simulink model "progetto_tesi_def"  (R2023b)
settings: Solver=ode1  StartTime=0.0  StopTime=inf  FixedStep=dt  RelTol=1e-3
values from neighbouring files (symbols this model uses):
  bias_acc = [0.1 , 0.1 , 0.1]    [model_params.m]
  degtoradianti = pi/180    (= 0.0174532925199)    [model_params.m]
  dt = 0.005    [model_params.m]
  gravity = -9.81007    [model_params.m]
  gyro_bias = gyro_bias_deg*degtoradianti    [model_params.m]
  Jhc = [0 0 0; 0 0 0; 0 0 0; 1 0 0; 0 1 0 ; 0 0 1]    [model_params.m]
  Jhe = [0 0 0 ; 0 0 l1 ; 0 -l1 0; 1 0 0; 0 1 0; 0 0 1]    [model_params.m]
  Jre = [0 0 0 1 0 0]'    [model_params.m]
  kc = 50    [model_params.m]
  noise_acc = 0.08 * gravity    (= -0.7848056)    [model_params.m]
  noise_gyro = 0.5* degtoradianti    (= 0.00872664625997)    [model_params.m]
  P_init = 1e-10 * eye(4)    [model_params.m]
  q_init = [1 0 0 0]'    [model_params.m]
  radiantitodeg = 180/pi    (= 57.2957795131)    [model_params.m]
undefined symbols (not defined in the file or in its folder): deg, m, s
libraries: qbmove_library x7, CP_library x2, dspstat3 x1, QB_pacer_lib x1, simulink x1
settings Model: Creator=ilari  LastModifiedBy=ilari

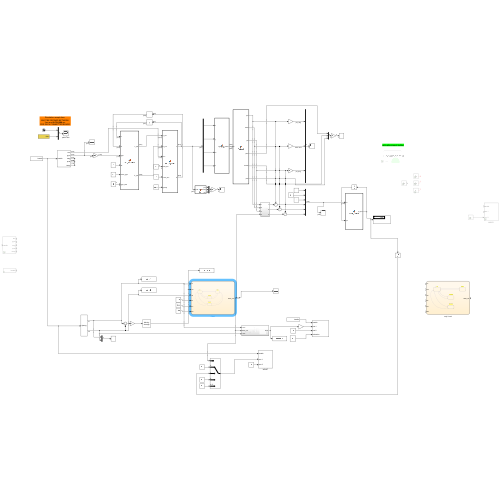
[thumbnail: Simulink's stored preview of the top-level diagram]
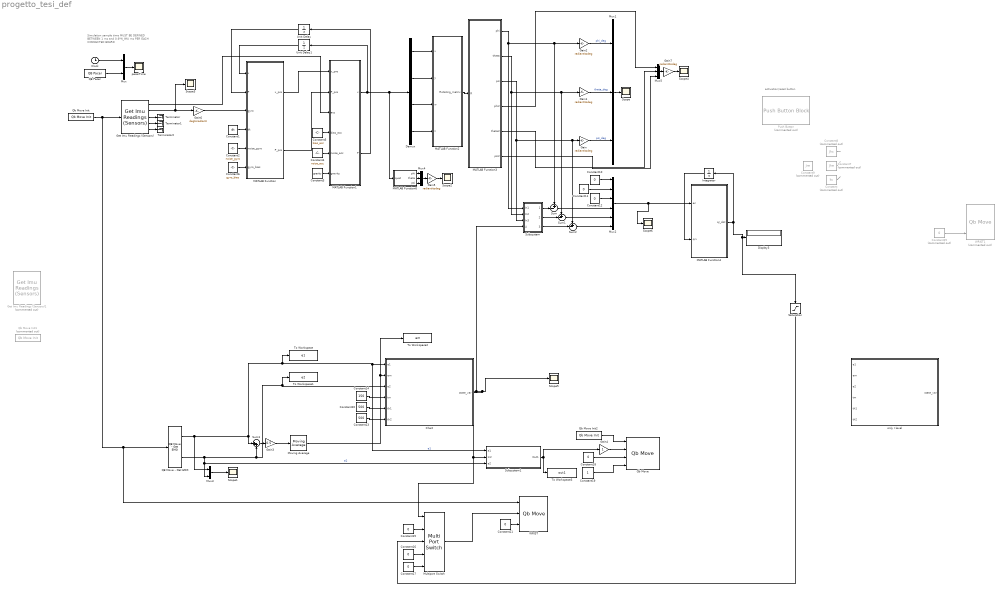
== system progetto_tesi_def ==
  note: activation/reset button
  note: Simulation sample time
      | MUST BE DEFINED BETWEEN
      | 1 ms and 0.6*N_IMU ms
      | PER EACH CONNECTED BOARD
  Chart : Stateflow chart  TreatAsAtomicUnit=on
  Clock : Clock
  Constant : Constant  Commented=on  Value=kc
  Constant1 : Constant  Value=dt
  Constant{10..12,15..18,21} (8 alike) : Constant  Value=0
  Constant13 : Constant  Value=500
  Constant14 : Constant  Value=150
  Constant19 : Constant
  Constant2 : Constant  Value=noise_gyro
  Constant20 : Constant  Value=500
  Constant25 : Constant  Commented=on  Value=0
  Constant3 : Constant  Value=gravity
  Constant4 : Constant  Value=noise_acc
  Constant5 : Constant  Value=bias_acc
  Constant6 : Constant  Value=gyro_bias
  Constant7 : Constant  Commented=on  Value=Jhe
  Constant8 : Constant  Commented=on  Value=Jhc
  Constant9 : Constant  Commented=on  Value=Jre
  Demux : Demux
  Display3 : Display
  Gain{,1..2,5,7} (5 alike) : Gain  Gain=radiantitodeg
  Gain3 : Gain  Gain=0.5
  Gain4 : Gain
  Gain6 : Gain  Gain=degtoradianti
  Get Imu Readings (Sensors) : CP_library/Get Imu Readings (Sensors)  ID=2  N_IMU=1  DAISY_CHAINING=off  ACC_UNITY=m/(s^2)  GYRO_UNITY=deg/s  MAG_UNITY=uT
      settings: SourceProductName=Centro Piaggio Library
  Get Imu Readings (Sensors)1 : CP_library/Get Imu Readings (Sensors)  Commented=on  ID=2  N_IMU=1  DAISY_CHAINING=off  ACC_UNITY=m/(s^2)  GYRO_UNITY=deg/s  MAG_UNITY=uT
      settings: SourceProductName=Centro Piaggio Library
  Integrator : Integrator
  MATLAB Function : MATLAB Function  TreatAsAtomicUnit=on
  MATLAB Function1 : MATLAB Function  TreatAsAtomicUnit=on
  MATLAB Function2 : MATLAB Function  TreatAsAtomicUnit=on
  MATLAB Function3 : MATLAB Function  TreatAsAtomicUnit=on
  MATLAB Function4 : MATLAB Function  TreatAsAtomicUnit=on
  MATLAB Function6 : MATLAB Function  TreatAsAtomicUnit=on
  Moving Average : dspstat3/Moving Average  Method=Sliding window  ForgettingFactorPort=off  SpecifyWindowLength=on  WindowLength=4  OverlapLength=3  AllowArbitraryInputLength=off  ForgettingFactor=0.9  SimulateUsing=Code generation
  Multiport Switch : MultiPortSwitch  DataPortOrder=Zero-based contiguous  Inputs=4  zeroidx=on  SaturateOnIntegerOverflow=off  InputSameDT=off
  Mux : Mux  Inputs=2
  Mux1 : Mux  Inputs=3
  Mux2 : Mux  Inputs=6
  Mux3 : Mux  Inputs=2
  Mux4 : Mux  Inputs=3
  Mux5 : Mux  Inputs=3
  Push Button : PushButtonBlock  Commented=on  Icon=Circle  IconAlignment=Right  IconColor=On  OffValue=0.000000
  QB Move - Get EMG : qbmove_library/QB Move - Get EMG  ID=2  DAISY_CHAINING=off
      settings: SourceProductName=Qb Move Library
  QB Pacer : QB_pacer_lib/QB Pacer  simTimePerRealTime=1
      settings: SourceProductName=QB Pacer
  Qb Move : qbmove_library/Qb Move  ID=1  ACTIVE_COMM_DIRECTIONS=Tx  CONTROL_MODE=Prime Movers Positions  DAISY_CHAINING=off  MAX_ANG=0  SW_LIMIT=inf  OFFSET=0  ACTIVATE=off  WDT=0.0  UNIT=TICK
      settings: LibrarySourceBlock=qbmove_library/qbmove  SourceProductName=Qb Move Library
  Qb Move Init : qbmove_library/Qb Move Init  NUMBER_OF_COM='COM9'  BAUD_RATE_COM=2000000
      settings: SourceProductName=Qb Move Library
  Qb Move Init1 : qbmove_library/Qb Move Init  Commented=on  NUMBER_OF_COM='COM9'  BAUD_RATE_COM=2000000
      settings: SourceProductName=Qb Move Library
  Qb Move Init2 : qbmove_library/Qb Move Init  NUMBER_OF_COM='COM7'  BAUD_RATE_COM=2000000
      settings: SourceProductName=Qb Move Library
  Saturation : Saturate  UpperLimit=100  LowerLimit=-100
  Scope{,1..6} (7 alike) : Scope
  Subsystem : Subsystem
  Subsystem1 : Subsystem
  Sum : Sum  Inputs=+-|
  Sum1 : Sum  Inputs=+-|
  Sum2 : Sum  Inputs=+-|
  Sum3 : Sum  Inputs=|++
  Terminator : Terminator
  Terminator1 : Terminator
  Terminator2 : Terminator
  To Workspace : ToWorkspace  VariableName=e1  SaveFormat=Timeseries  SampleTime=-1
  To Workspace1 : ToWorkspace  VariableName=e2  SaveFormat=Timeseries  SampleTime=-1
  To Workspace2 : ToWorkspace  VariableName=em  SaveFormat=Timeseries  SampleTime=-1
  To Workspace3 : ToWorkspace  VariableName=out1  SaveFormat=Timeseries  SampleTime=-1
  Unit Delay : UnitDelay  InitialCondition=P_init  SampleTime=-1  HasFrameUpgradeWarning=on
  Unit Delay1 : UnitDelay  InitialCondition=q_init  SampleTime=-1  HasFrameUpgradeWarning=on
  WRIST : qbmove_library/Qb Move  ID=2  ACTIVE_COMM_DIRECTIONS=Tx  CONTROL_MODE=Prime Movers Positions  DAISY_CHAINING=off  MAX_ANG=0  SW_LIMIT=inf  OFFSET=0  ACTIVATE=on  WDT=0.0  UNIT=TICK
      settings: SourceProductName=Qb Move Library
  WRIST1 : qbmove_library/Qb Move  Commented=on  ID=2  ACTIVE_COMM_DIRECTIONS=Tx  CONTROL_MODE=Prime Movers Positions  DAISY_CHAINING=off  MAX_ANG=0  SW_LIMIT=inf  OFFSET=0  ACTIVATE=on  WDT=0.0  UNIT=TICK
      settings: SourceProductName=Qb Move Library
  only I level : Stateflow chart  TreatAsAtomicUnit=on
  pacerTime : Scope
  wires:
  Clock/1 -> Mux/1
  Mux/1 -> pacerTime/1
  QB Pacer/1 -> Mux/2
  Qb Move Init/1 -> WRIST/1, QB Move - Get EMG/1, Get Imu Readings (Sensors)/1
  Get Imu Readings (Sensors)/5 -> Terminator2/1
  Get Imu Readings (Sensors)/4 -> Terminator1/1
  Get Imu Readings (Sensors)/3 -> Terminator/1
  Get Imu Readings (Sensors)/2 -> Scope3/1, Gain6/1
  MATLAB Function/1(x_pre) -> MATLAB Function1/1(x_pre)
  MATLAB Function/2(P_pre) -> MATLAB Function1/2(P_pre)
  Get Imu Readings (Sensors)/1 -> MATLAB Function1/3(acc)
  MATLAB Function1/1(x) -> MATLAB Function6/1(quat), Demux/1, Unit Delay1/1
  Unit Delay1/1 -> MATLAB Function/1(x)
  MATLAB Function1/2(P) -> Unit Delay/1
  Unit Delay/1 -> MATLAB Function/2(P)
  Demux/1 -> MATLAB Function2/1(x)
  Demux/2 -> MATLAB Function2/2(y)
  Demux/3 -> MATLAB Function2/3(w)
  Demux/4 -> MATLAB Function2/4(z)
  MATLAB Function2/1(Rotating_matrix) -> MATLAB Function3/1(R)
  MATLAB Function3/1(phi) -> Subsystem/1(In1), Gain2/1, Sum/1
  MATLAB Function3/2(theta) -> Subsystem/2(In2), Sum1/1, Gain1/1
  MATLAB Function3/3(psi) -> Subsystem/3(In3), Sum2/1, Gain/1
  Gain2/1 -> Mux1/1  "phi_deg"
  Gain1/1 -> Mux1/2  "theta_deg"
  Gain/1 -> Mux1/3  "psi_deg"
  Mux1/1 -> Scope/1
  Gain6/1 -> MATLAB Function/3(gyro)
  Constant1/1 -> MATLAB Function/4(dt)
  Constant2/1 -> MATLAB Function/5(noise_gyro)
  Constant3/1 -> MATLAB Function1/6(gravity)
  Constant4/1 -> MATLAB Function1/5(noise_acc)
  Constant5/1 -> MATLAB Function1/4(bias_acc)
  Constant6/1 -> MATLAB Function/6(gyro_bias)
  Constant8/1 -> ?
  Constant7/1 -> ?
  Constant/1 -> ?
  Subsystem/1(Output) -> Sum/2
  Subsystem/3(Output2) -> Sum2/2
  Subsystem/2(Output1) -> Sum1/2
  Sum/1 -> Mux2/4
  Sum1/1 -> Mux2/5
  Sum2/1 -> Mux2/6
  Constant10/1 -> Mux2/1
  Constant12/1 -> Mux2/3
  Constant11/1 -> Mux2/2
  Mux2/1 -> Scope6/1, MATLAB Function4/1(ec)
  Integrator/1 -> MATLAB Function4/2(qrx)
  Constant25/1 -> WRIST1/3
  MATLAB Function6/1(phi) -> Mux4/1
  MATLAB Function6/2(theta) -> Mux4/2
  MATLAB Function6/3(psi) -> Mux4/3
  Mux4/1 -> Gain5/1
  Gain5/1 -> Scope2/1
  Mux5/1 -> Gain7/1
  Gain7/1 -> Scope4/1
  MATLAB Function3/4(phi2) -> Mux5/1
  MATLAB Function3/5(theta2) -> Mux5/2
  MATLAB Function3/6(psi2) -> Mux5/3
  Chart/1(state_var) -> Multiport Switch/1, Subsystem1/2(In2), Subsystem/4(Input), Scope5/1
  Constant20/1 -> Chart/5(th1)
  Constant14/1 -> Chart/4(tm)
  Mux3/1 -> Scope1/1
  Moving Average/1 -> Chart/2(em), To Workspace2/1
  QB Move - Get EMG/2 -> Mux3/2, Subsystem1/3(e2), Chart/3(e2), To Workspace1/1, Sum3/2  "e2"
  QB Move - Get EMG/1 -> Mux3/1, Sum3/1, To Workspace/1, Chart/1(e1), Subsystem1/1(e1)  "e1"
  Constant13/1 -> Chart/6(th2)
  Multiport Switch/1 -> WRIST/2
  Qb Move Init2/1 -> Qb Move/1
  Subsystem1/1(Out1) -> To Workspace3/1, Gain4/1
  Gain3/1 -> Moving Average/1
  MATLAB Function4/1(qr_dot) -> Integrator/1, Saturation/1, Display3/1
  Sum3/1 -> Gain3/1
  Constant15/1 -> Multiport Switch/2
  Constant17/1 -> Multiport Switch/5
  Constant18/1 -> Qb Move/3
  Constant21/1 -> WRIST/3
  Constant16/1 -> Multiport Switch/4
  Constant19/1 -> Qb Move/4
  Saturation/1 -> Multiport Switch/3
  Gain4/1 -> Qb Move/2

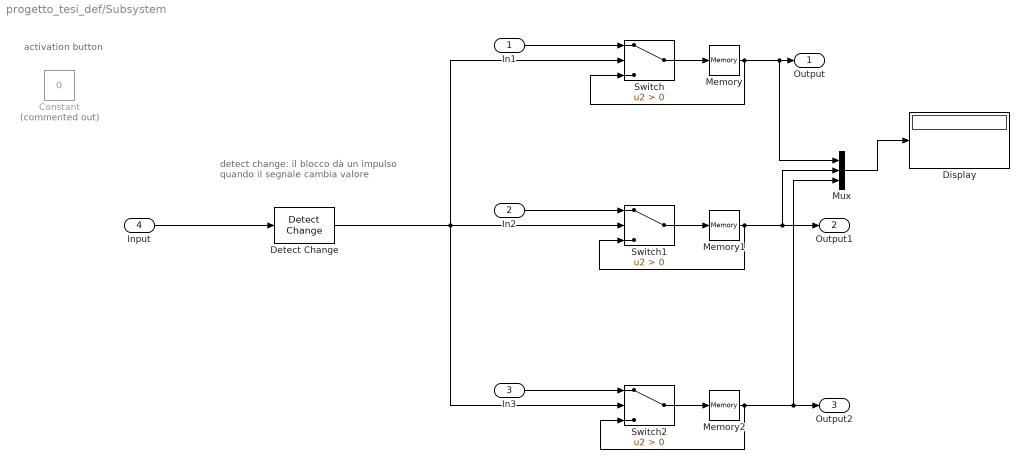
== system progetto_tesi_def/Subsystem ==
  note: detect change: il blocco dà un impulso
      |  quando il segnale cambia valore
  note: activation button
  In1 : Inport
  In2 : Inport  Port=2
  In3 : Inport  Port=3
  Input : Inport  Port=4
  Constant : Constant  Commented=on  Value=0
  Detect Change : simulink/Logic and Bit Operations/Detect Change  vinit=0  OutDataTypeStr=boolean
  Display : Display
  Memory : Memory
  Memory1 : Memory
  Memory2 : Memory
  Mux : Mux  Inputs=3
  Switch : Switch  Criteria=u2 > Threshold  SaturateOnIntegerOverflow=off  InputSameDT=off
  Switch1 : Switch  Criteria=u2 > Threshold  SaturateOnIntegerOverflow=off  InputSameDT=off
  Switch2 : Switch  Criteria=u2 > Threshold  SaturateOnIntegerOverflow=off  InputSameDT=off
  Output : Outport
  Output1 : Outport  Port=2
  Output2 : Outport  Port=3
  wires:
  Memory/1 -> Switch/3, Mux/1, Output/1
  Switch1/1 -> Memory1/1
  Memory1/1 -> Switch1/3, Output1/1, Mux/2
  Switch2/1 -> Memory2/1
  Memory2/1 -> Switch2/3, Output2/1, Mux/3
  Switch/1 -> Memory/1
  In1/1 -> Switch/1
  In2/1 -> Switch1/1
  In3/1 -> Switch2/1
  Detect Change/1 -> Switch/2, Switch2/2, Switch1/2
  Input/1 -> Detect Change/1
  Mux/1 -> Display/1

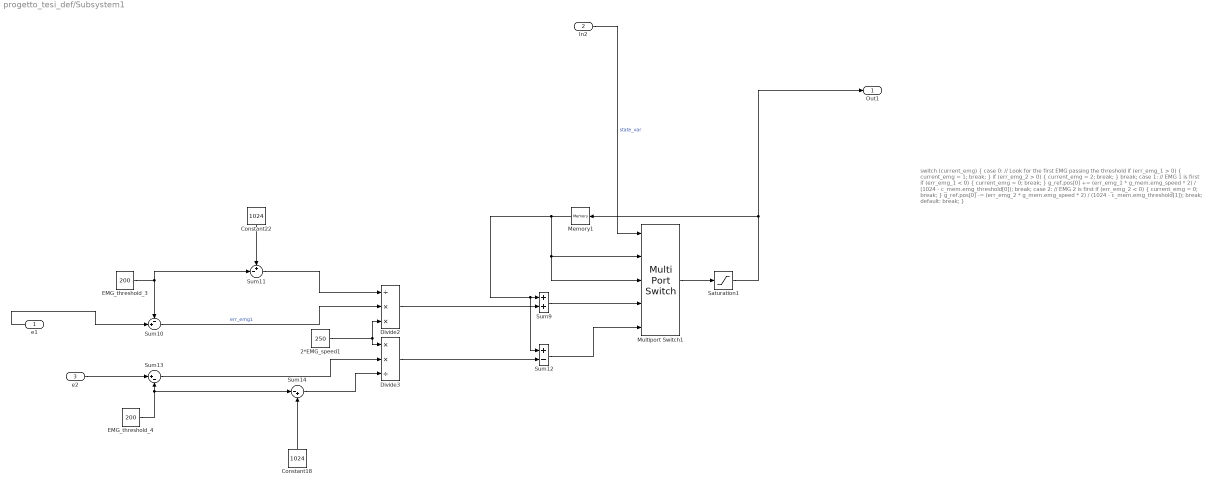
== system progetto_tesi_def/Subsystem1 ==
  note: switch (current_emg) {
      | case 0:
      | // Look for the first EMG passing the threshold
      | if (err_emg_1 > 0) {
      | current_emg = 1;
      | break;
      | }
      | if (err_emg_2 > 0) {
      | current_emg = 2;
      | break;
      | }
      | break;
      |
      | case 1:
      | // EMG 1 is first
      | if (err_emg_1 < 0) {
      | current_emg = 0;
      | break;
      | }
      | g_ref.pos[0] += (err_emg_1 * g_mem.emg_speed * 2) / (1024 - c_mem.emg_threshold[0]);
      | break;
      |
      | case 2:
      | // EMG 2 is first
      | if (err_emg_2 < 0) {
      | current_emg = 0;
      | break;
      | }
      | g_ref.pos[0] -= (err_emg_2 * g_mem.emg_speed * 2) / (1024 - c_mem.emg_threshold[1]);
      | break;
      |
      | default:
      | break;
      | }
  e1 : Inport
  In2 : Inport  Port=2
  e2 : Inport  Port=3
  2*EMG_speed1 : Constant  Value=250
  Constant18 : Constant  Value=1024
  Constant22 : Constant  Value=1024
  Divide2 : Product  Inputs=/**
  Divide3 : Product  Inputs=**/
  EMG_threshold_3 : Constant  Value=200
  EMG_threshold_4 : Constant  Value=200
  Memory1 : Memory
  Multiport Switch1 : MultiPortSwitch  DataPortOrder=Zero-based contiguous  Inputs=4  zeroidx=on  SaturateOnIntegerOverflow=off  InputSameDT=off
  Saturation1 : Saturate  UpperLimit=17500  LowerLimit=0
  Sum10 : Sum  Inputs=-+|
  Sum11 : Sum  Inputs=+-|
  Sum12 : Sum  Inputs=+-
  Sum13 : Sum  Inputs=|+-
  Sum14 : Sum  Inputs=|-+
  Sum9 : Sum
  Out1 : Outport
  wires:
  Multiport Switch1/1 -> Saturation1/1
  Memory1/1 -> Multiport Switch1/2, Multiport Switch1/3, Sum12/1, Sum9/1
  e1/1 -> Sum10/2
  Sum11/1 -> Divide2/1
  Sum9/1 -> Multiport Switch1/4
  Saturation1/1 -> Out1/1, Memory1/1
  Divide2/1 -> Sum9/2
  Divide3/1 -> Sum12/2
  Sum14/1 -> Divide3/3
  EMG_threshold_3/1 -> Sum11/2, Sum10/1
  EMG_threshold_4/1 -> Sum14/1, Sum13/2
  Constant18/1 -> Sum14/2
  2*EMG_speed1/1 -> Divide3/1, Divide2/3
  Sum13/1 -> Divide3/2
  e2/1 -> Sum13/1
  Sum12/1 -> Multiport Switch1/5
  Sum10/1 -> Divide2/2  "err_emg1"
  Constant22/1 -> Sum11/1
  In2/1 -> Multiport Switch1/1  "state_var"

== stateflow chart progetto_tesi_def/only I level ==
  note: rest
  note: polso on
  state state0
    entry: state_var = 0;
  state state1
    entry: state_var=1;
  note: mano chiusa
  state state2
    entry: state_var=2;
  note: mano aperta
  state state3
    entry: state_var=3;
  (default) -> state0
  state0 -> state1 [order 1] : [em>tm && e1<th1 && e2<th2 && after(2, sec)]
  state1 -> state0 : [em<tm && after(2, sec)]
  state3 -> state0 : [em<tm && e2<th2 && after(2, sec)]
  state0 -> state3 [order 3] : [em>tm && e2>th2 && after(2, sec)]
  state0 -> state2 [order 2] : [em>tm && e1>th1 && after(2, sec)]
  state2 -> state0 : [em<tm && e1<th1 && after(2, sec)]
  data: e1 input; em input size=1; e2 input; tm input; th1 input; state_var output; th2 input

== matlab function progetto_tesi_def/MATLAB Function6 ==
  data: quat input; phi output; theta output; psi output
function [phi, theta , psi] = fcn(quat)

q0 = quat(1);
q1 = quat(2);
q2 = quat(3);
q3 = quat(4);

phi = atan2(2*(q2*q3 + q0*q1), q0^2 -q1^2 -q2^2 +q3^2);
theta = -asin(2*(q1*q3 -q0*q2));
psi = atan2(2*(q1*q2 + q0*q3), q0^2 + q1^2 -q2^2 -q3^2);

end

== matlab function progetto_tesi_def/MATLAB Function1 ==
  data: x_pre input; x output size=[4 1]; P_pre input; acc input; bias_acc input size=[1 3]; noise_acc input; gravity input; P output
function [x , P] = EKF_update(x_pre , P_pre , acc  , bias_acc , noise_acc,  gravity)

% Inizializzazione variabili di output
x = x_pre;
P = P_pre;

%correzione delle letture
acc = acc - bias_acc;
%mag = mag - bias_mag;

%Update accelerometro
if norm(acc) ~= 0
    acc_norm = acc'/norm(acc);
else
    acc_norm = acc'; %[3x1]
end

%utilizzo formula gravità come modello di osservazione

acc_prediction = [ 2*(x_pre(2)*x_pre(4)-x_pre(1)*x_pre(3));
                   2*(x_pre(3)*x_pre(4)+x_pre(1)*x_pre(2));
                   x_pre(1)^2-x_pre(2)^2-x_pre(3)^2+x_pre(4)^2]; %[3x1]

%calcolo del residuo (innovazione)
y_acc = acc_norm - acc_prediction;  %[3x1]

% derivo modello di osservazione per ottenere la matrice H
H_acc =   2 * [-x_pre(3)    x_pre(4)    -x_pre(1)   x_pre(2); 
            x_pre(2)    x_pre(1)     x_pre(4)   x_pre(3); 
            x_pre(1)   -x_pre(2)    -x_pre(3)   x_pre(4)]; %[3x4]

% Rumore di misura R
if norm(acc) ~= 0 
    R_acc_internal = (noise_acc / norm(acc))^2 * eye(3);
    R_acc_external = (1-gravity/norm(acc))^2 * eye(3);
    R_acc = R_acc_internal + R_acc_external;
else 
    R_acc = eye(3);
end

%  fase di Update accelerometro

S_acc = H_acc * P_pre * H_acc' + R_acc; %[3x3]
K_acc = P_pre * H_acc' / S_acc; %[4x3]
x = x_pre + K_acc * y_acc; %[4x1]
P = (eye(4) - K_acc * H_acc) * P_pre; %[4x4]

% %% Update magnetometro
% 
% if norm(mag) ~= 0
%     mag_norm = mag'/norm(mag);
% else
%     mag_norm = mag'; %[3x1]
% end
% 
% mag_prediction = [ 2*(x_pre(2)*x_pre(4)+x_pre(1)*x_pre(3));
%                    2*(x_pre(3)*x_pre(4)-x_pre(1)*x_pre(2));
%                    x_pre(1)^2-x_pre(2)^2-x_pre(3)^2+x_pre(4)^2]; %[3x1]
% 
% y_mag = mag_norm - mag_prediction;  %[3x1]
% 
% H_mag = 2 * [ x_pre(3)    x_pre(4)     x_pre(1)    x_pre(2);
%              -x_pre(2)    x_pre(1)    -x_pre(4)    x_pre(3);
%               x_pre(1)   -x_pre(2)    -x_pre(3)    x_pre(4)]; %[3x4]
% 
% R_mag = eye(3);
% 
% if norm(mag) ~= 0
%     R_mag = (noise_mag / norm(mag))^2 * eye(3);
% end
% 
% S_mag = H_mag * P * H_mag' + R_mag; %[3x3]
% K_mag = P * H_mag' / S_mag; %[4x3]
% x = x + K_mag * y_mag; %[4x1]
% P = (eye(4) - K_mag * H_mag) * P;


if norm(x) ~= 0
    x = x/norm(x);
else


end

== matlab function progetto_tesi_def/MATLAB Function ==
  data: x input size=[4 1]; x_pre output; P input; gyro input; P_pre output; dt input; noise_gyro input; gyro_bias input
function [x_pre, P_pre] = EKF_prediction(x, P, gyro, dt, noise_gyro, gyro_bias)

    % x: stato corrente [ q0 q1 q2 q3 bx by bz] [7x1]
    %pre = predetto

    % P: matrice covarianza dello stato

    % z: misurazione (accelerometro e magnetometro)

    % gyro (u) ingresso di controllo (dati del giroscopio) [wx wy wz] [p q r]

    % Q: covarianza del rumore di processo

    % R: covarianza del rumore di misura

   

   %% STATO
       
    %       |   q0    |
    %       |   q1    |
    %  x =  |   q2    |
    %       |   q3    |

    %% Predizione

   %   x(k+1) ~= x(k) + f(x(k),0)*dt
   % 
   % q0 = state_hat(1);
   % q1 = state_hat(2);
   % q2 = state_hat(3);
   % q3 = state_hat(4);

   % correggo le misure di giroscopio 

   wx = gyro(1) - gyro_bias(1);
   wy = gyro(2) - gyro_bias(2);
   wz = gyro(3) - gyro_bias(3);

   % wx = gyro(1);
   % wy = gyro(2);
   % wz = gyro(3);


   
   Omega =[ 0   -wx  -wy  -wz;
            wx   0    wz   -wy; 
            wy  -wz   0     wx;
            wz   wy  -wx    0  ];


   F = eye(4) + dt * 0.5 * Omega ;



   % dot_matrix = [0     -(wx-bx)     -(wy-by)    -(wz-bz)   0 0 0;
   %              (wx-bx)     0        (wz-bz)    -(wy-by)   0 0 0;
   %              (wy-by) -(wz-bz)        0        (wx-bz)   0 0 0;
   %              (wz-bz)  (wy-by)     -(wx-bx)       0      0 0 0;
   %                0         0            0          0      0 0 0;
   %                0         0            0          0      0 0 0;
   %                0         0            0          0      0 0 0]; %[7x7]

  
  % state_hat_pre = state_hat + 0.5*dt*dot_matrix*state_hat  %stato predetto
  
  
  % Compute the process noise Q %capire da dove viene la formula

    G = [-x(2)  -x(3)  -x(4); 
          x(1)  -x(4)   x(3); 
          x(4)   x(1)  -x(2); 
         -x(3)   x(2)   x(1)] / 2;

    Q = (noise_gyro * dt)^2 * (G * G');
    
    % Propagate the state and covariance
    x_pre = F * x;
    x_pre = x_pre / norm(x_pre);    % Normalize the quaternion
    P_pre = F * P * F' + Q;
    

end

== matlab function progetto_tesi_def/MATLAB Function2 ==
  data: x input; Rotating_matrix output; y input; w input; z input
function Rotating_matrix = Quat2rot(x , y , w ,z)

Rotating_matrix = [(1 - 2*(y^2 + z^2)) , 2*(x*y - w*z) , 2*(w*y + x*z);
                    2*(x*y + w*z) , (1 - 2*(x^2 + z^2)) , 2*(y*z - w*x);
                    2*(x*z - w*y) , 2*(w*x + y*z) , (1 - 2*(x^2 + y^2))];
end

== matlab function progetto_tesi_def/MATLAB Function3 ==
  data: R input; phi output; theta output; psi output; phi2 output; theta2 output; psi2 output
function [ phi , theta , psi, phi2, theta2 , psi2]  = Rot2eul(R)


% Verifico che la matrice R sia 3x3

assert(all(size(R) == [3 3]), 'La matrice di rotazione deve essere 3x3');

% Calcolo dell'angolo 

R31 = R(3,1);

if R31 ~= 1 && R31 ~= -1

    theta1 = -asin(R31);
    theta2 = pi - theta1;

    %psi1 = atan2(R(3,2) / cos(theta1), R(3,3) / cos(theta1));
    psi1 = atan2(R(3,2), R(3,3));
    psi2 = atan2(R(3,2) / cos(theta2), R(3,3) / cos(theta2));

    % phi1 = atan2(R(2,1) / cos(theta1), R(1,1) /cos(theta1));
    phi1 = atan2(R(2,1), R(1,1));
    phi2 = atan2(R(2,1) / cos(theta2), R(1,1) / cos(theta2));

else

   phi1 = 0;
   phi2 = 0;

   if R31 == 1
       theta1 = pi/2;
       theta2 = pi/2;
       psi1 = phi1 + atan2(R(1,2), R(1,3));
       psi2 = phi1 + atan2(R(1,2), R(1,3));
   else
       theta1 = - pi/2;
       theta2 = - pi/2;
       psi1 = -phi1 + atan2(-R(1,2), -R(1,3));
       psi2 = -phi1 + atan2(-R(1,2), -R(1,3));
   end
end


% Seleziono una soluzione
psi = psi1;  % o psi2
theta = theta1;  % o theta2
phi = phi1;  % o phi2

== matlab function progetto_tesi_def/MATLAB Function4 ==
  data: qr_dot output; ec input size=[1 6]; qrx input
% function qr_dot = wrist_control(ec, Jre , Jhc , Jhe , kc)
% ec = ec'; %deve essere 6x1
% Jre_i = pinv(Jre);
% Jhe_i = pinv(Jhe);
% qr_dot = -Jre_i*(pinv(Jhc*Jhe_i))*kc*ec ;
% 
% end

function qr_dot = wrist_control(ec, qrx)

ec = ec';
alpha = ec(4); %phi
beta = ec(5);  %theta
gamma = ec(6); %psi
kc = 100;
l1=0.3; %[m]
lw = 0.1; %[m]
Rxyz =[cos(beta)*cos(gamma) , (sin(alpha)*sin(beta)*cos(gamma))-(cos(alpha)*sin(gamma)), (cos(alpha)*sin(beta)*cos(gamma))+(sin(alpha)*sin(gamma));
       cos(beta)*sin(gamma) , (sin(alpha)*sin(beta)*sin(gamma))+(cos(alpha)*cos(gamma)), (cos(alpha)*sin(beta)*sin(gamma))-(sin(alpha)*cos(gamma));
       -sin(beta)           , sin(alpha)*cos(beta)                                     ,  cos(alpha)*cos(beta)                                     ];  

Rx_qrx = [1 0 0; 0 cos(qrx) -sin(qrx); 0 sin(qrx) cos(qrx)];

Rxyzx = Rxyz*Rx_qrx;

vector_p = [-l1 0 0]';
vector_p_tras = Rxyz*vector_p + Rxyzx*[-lw ; 0 ; 0];
z1 = Rxyzx(:,1);
z2 = Rxyzx(:,2);
z3 = Rxyzx(:,3);

Jrc = [0 0 0 0 0 0]';
Jhc = [zeros(3,3); Rxyz];
Jre = [0;0;0;z1];
Jhe = [cross(z1,vector_p_tras) , cross(z2,vector_p_tras) , cross(z1,vector_p_tras); z1, z2, z3];

Jre_i = pinv(Jre);
Jhe_i = pinv(Jhe);
K=-Jre_i*(pinv(Jhc*Jhe_i))*kc;
qr_dot = -Jre_i*(pinv(Jhc*Jhe_i))*kc*ec;

== stateflow chart progetto_tesi_def/Chart ==
  note: rest
  note: polso on
  state state0
    entry: state_var = 0;
  state state1
    entry: state_var=1;
  note: mano chiusa
  state state2
    entry: state_var=2;
  note: mano aperta
  state state3
    entry: state_var=3;
  (default) -> state0
  state0 -> state1 [order 1] : [em>tm & e1<th1 & e2<th2 & after(2,sec)]
  state1 -> state0 [order 1] : [em<tm & after(2,sec)]
  state1 -> state3 [order 2] : [em>tm & e2>th2 & after(2,sec)]
  state3 -> state0 : [em<tm & e2<th2]
  state3 -> state1 [commented out] : [em>tm & e2<th2]
  state0 -> state3 [order 3] : [em>tm & e2>th2]
  state0 -> state2 [order 2] : [em<tm & e1>th1]
  state2 -> state0 : [em<tm & e1<th1]
  state2 -> state1 [commented out] : [em>tm &e1<th1]
  state1 -> state2 [order 3] : [em>tm & e1>th1 & after(2,sec)]
  data: e1 input; em input size=1; e2 input; tm input; th1 input; state_var output; th2 input
